simulink model "ysw3_15"  (R2014a)
settings: Solver=ode45  StartTime=0.0  StopTime=10.0  RelTol=1e-3
settings Model: Creator=Administrator  LastModifiedBy=Administrator

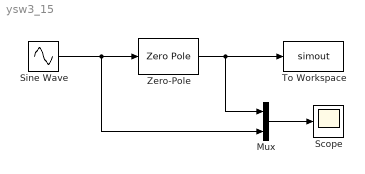
== system ysw3_15 ==
  Mux : Mux  Inputs=2
  Scope : Scope
      settings: TimeRange=10
  Sine Wave : Sin  SampleTime=0
  To Workspace : ToWorkspace  VariableName=simout  SaveFormat=Timeseries  SampleTime=-1
  Zero-Pole : ZeroPole  Poles=[0 -1]
  wires:
  Mux/1 -> Scope/1
  Sine Wave/1 -> Mux/2, Zero-Pole/1
  Zero-Pole/1 -> Mux/1, To Workspace/1
